simulink model "CVD"  (R2013a)
settings: Solver=ode45  StartTime=0.0  StopTime=1  RelTol=1e-3
settings Model: Creator=Max Simmonds  LastModifiedBy=Max Simmonds

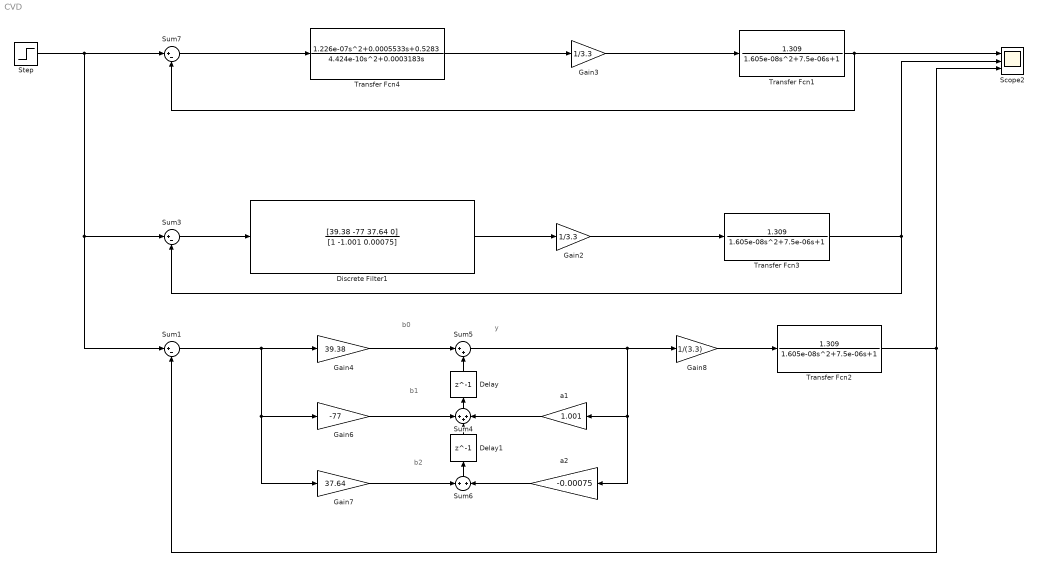
== system CVD ==
  note: y
  note: b2
  note: b1
  note: b0
  Delay : Delay  DelayLength=1  InitialCondition=0  SampleTime=1e-5
  Delay1 : Delay  DelayLength=1  InitialCondition=0  SampleTime=1e-5
  Discrete Filter1 : DiscreteFilter  Numerator=[39.38 -77 37.64 0]  Denominator=[1 -1.001 0.00075]  SampleTime=1e-5
  Gain2 : Gain  Gain=1/3.3
  Gain3 : Gain  Gain=1/3.3
  Gain4 : Gain  Gain=39.38  SampleTime=1e-5
  Gain6 : Gain  Gain=-77  SampleTime=1e-5
  Gain7 : Gain  Gain=37.64  SampleTime=1e-5
  Gain8 : Gain  Gain=1/(3.3)
  Scope2 : Scope  NumInputPorts=3
      settings: TimeRange=0.003173749327595482  YMin=1.79875~-5~-5  YMax=1.80125~5~5  SaveName=ScopeData2
  Step : Step  Time=0.5  After=5  SampleTime=0
  Sum1 : Sum  Inputs=|+-  SampleTime=1e-5
  Sum3 : Sum  Inputs=|+-  SampleTime=1e-5
  Sum4 : Sum  Inputs=+++  SampleTime=1e-5
  Sum5 : Sum  Inputs=|++  SampleTime=1e-5
  Sum6 : Sum  SampleTime=1e-5
  Sum7 : Sum  Inputs=|+-  SampleTime=1e-5
  Transfer Fcn1 : TransferFcn  Numerator=[1.309]  Denominator=[1.605e-08 7.5e-06 1]
  Transfer Fcn2 : TransferFcn  Numerator=[1.309]  Denominator=[1.605e-08 7.5e-06 1]
  Transfer Fcn3 : TransferFcn  Numerator=[1.309]  Denominator=[1.605e-08 7.5e-06 1]
  Transfer Fcn4 : TransferFcn  Numerator=[1.226e-07 0.0005533 0.5283]  Denominator=[ 4.424e-10 0.0003183 0]
  a1 : Gain  Gain=1.001  SampleTime=1e-5
  a2 : Gain  Gain=-0.00075  SampleTime=1e-5
  wires:
  Step/1 -> Sum1/1, Sum3/1, Sum7/1
  Sum3/1 -> Discrete Filter1/1
  Discrete Filter1/1 -> Gain2/1
  Gain2/1 -> Transfer Fcn3/1
  Transfer Fcn3/1 -> Scope2/2, Sum3/2
  a1/1 -> Sum4/3
  Gain6/1 -> Sum4/1
  a2/1 -> Sum6/2
  Gain7/1 -> Sum6/1
  Sum1/1 -> Gain7/1, Gain6/1, Gain4/1
  Sum4/1 -> Delay/1
  Delay1/1 -> Sum4/2
  Sum6/1 -> Delay1/1
  Sum5/1 -> Gain8/1, a2/1, a1/1
  Delay/1 -> Sum5/2
  Gain4/1 -> Sum5/1
  Gain8/1 -> Transfer Fcn2/1
  Transfer Fcn2/1 -> Sum1/2, Scope2/3
  Sum7/1 -> Transfer Fcn4/1
  Transfer Fcn4/1 -> Gain3/1
  Gain3/1 -> Transfer Fcn1/1
  Transfer Fcn1/1 -> Scope2/1, Sum7/2
